simulink model "kkadai11"  (R2021b)
settings: Solver=VariableStepAuto  StartTime=0.0  StopTime=100  RelTol=1e-3
settings Model: Creator=tomotomo  LastModifiedBy=tomotomo

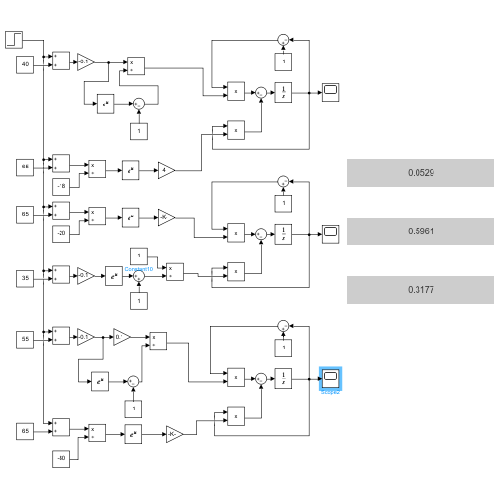
[thumbnail: Simulink's stored preview of the top-level diagram]
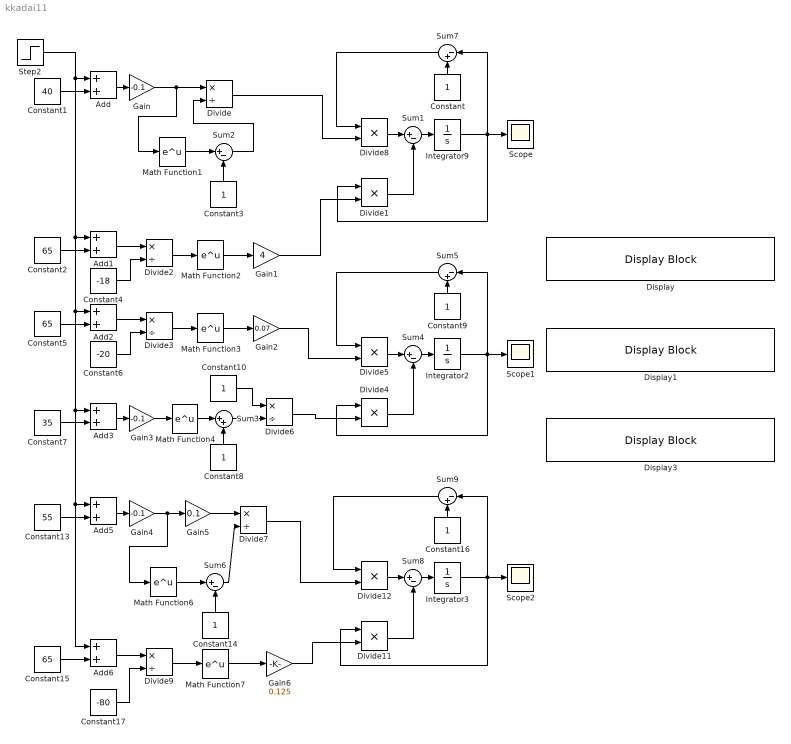
== system kkadai11 ==
  Add{,1..3,5..6} (6 alike) : Sum
  Constant{,3,8..10,14,16} (7 alike) : Constant
  Constant1 : Constant  Value=40
  Constant13 : Constant  Value=55
  Constant15 : Constant  Value=65
  Constant17 : Constant  Value=-80
  Constant2 : Constant  Value=65
  Constant4 : Constant  Value=-18
  Constant5 : Constant  Value=65
  Constant6 : Constant  Value=-20
  Constant7 : Constant  Value=35
  Display : DisplayBlock  LabelPosition=Hide  Format=short  Transparency=1
  Display1 : DisplayBlock  LabelPosition=Hide  Format=short  Transparency=1
  Display3 : DisplayBlock  LabelPosition=Hide  Format=short  Transparency=1
  Divide{,2..3,6..7,9} (6 alike) : Product  Inputs=*/
  Divide{1,4..5,8,11..12} (6 alike) : Product  Inputs=**
  Gain : Gain  Gain=-0.1
  Gain1 : Gain  Gain=4
  Gain2 : Gain  Gain=0.07
  Gain3 : Gain  Gain=-0.1
  Gain4 : Gain  Gain=-0.1
  Gain5 : Gain  Gain=0.1
  Gain6 : Gain  Gain=0.125
  Integrator2 : Integrator
  Integrator3 : Integrator
  Integrator9 : Integrator
  Math Function{1..4,6..7} (6 alike) : Math  SaturateOnIntegerOverflow=on
  Scope : Scope
  Scope1 : Scope
  Scope2 : Scope
  Step2 : Step  Time=2  Before=-65  After=-65  SampleTime=0
  Sum{1..2,4,6,8} (5 alike) : Sum  Inputs=|+-
  Sum3 : Sum  Inputs=|++
  Sum5 : Sum  Inputs=|-+
  Sum7 : Sum  Inputs=|-+
  Sum9 : Sum  Inputs=|-+
  wires:
  Constant15/1 -> Add6/2
  Math Function7/1 -> Gain6/1
  Divide/1 -> Divide8/2
  Sum6/1 -> Divide7/2
  Constant2/1 -> Add1/2
  Divide11/1 -> Sum8/2
  Sum9/1 -> Divide12/1
  Constant16/1 -> Sum9/2
  Sum8/1 -> Integrator3/1
  Add6/1 -> Divide9/1
  Divide12/1 -> Sum8/1
  Constant14/1 -> Sum6/2
  Math Function6/1 -> Sum6/1
  Math Function1/1 -> Sum2/1
  Gain6/1 -> Divide11/2
  Constant13/1 -> Add5/2
  Sum1/1 -> Integrator9/1
  Sum2/1 -> Divide/2
  Constant4/1 -> Divide2/2
  Constant/1 -> Sum7/2
  Sum7/1 -> Divide8/1
  Constant1/1 -> Add/2
  Add1/1 -> Divide2/1
  Math Function2/1 -> Gain1/1
  Gain1/1 -> Divide1/2
  Divide2/1 -> Math Function2/1
  Constant5/1 -> Add2/2
  Math Function3/1 -> Gain2/1
  Divide3/1 -> Math Function3/1
  Add2/1 -> Divide3/1
  Divide1/1 -> Sum1/2
  Add5/1 -> Gain4/1
  Gain3/1 -> Math Function4/1
  Integrator9/1 -> Sum7/1, Scope/1, Divide1/1
  Add3/1 -> Gain3/1
  Divide8/1 -> Sum1/1
  Constant8/1 -> Sum3/2
  Constant6/1 -> Divide3/2
  Constant7/1 -> Add3/2
  Gain2/1 -> Divide5/2
  Gain/1 -> Divide/1, Math Function1/1
  Constant17/1 -> Divide9/2
  Constant3/1 -> Sum2/2
  Divide9/1 -> Math Function7/1
  Sum5/1 -> Divide5/1
  Divide4/1 -> Sum4/2
  Divide5/1 -> Sum4/1
  Sum4/1 -> Integrator2/1
  Constant9/1 -> Sum5/2
  Add/1 -> Gain/1
  Math Function4/1 -> Sum3/1
  Gain5/1 -> Divide7/1
  Divide7/1 -> Divide12/2
  Gain4/1 -> Gain5/1, Math Function6/1
  Step2/1 -> Add6/1, Add5/1, Add3/1, Add2/1, Add1/1, Add/1
  Integrator2/1 -> Scope1/1, Divide4/1, Sum5/1
  Integrator3/1 -> Scope2/1, Divide11/1, Sum9/1
  Sum3/1 -> Divide6/2
  Divide6/1 -> Divide4/2
  Constant10/1 -> Divide6/1
